simulink model "TestCinematiqueNew"  (Simulink 6.5)
settings: Solver=ode45  StartTime=0.0  StopTime=10.0  RelTol=1e-3
undefined symbols (not defined in the file): EngineSpeedTest, EngineSpeedTimeTest, x
settings Model: Creator=a030141  LastModifiedBy=Zeus
settings DataIOCC: SignalLoggingName=sigsOut
settings DebuggingCC: SolverPrmCheckMsg=none  MultiTaskDSMMsg=warning  MultiTaskCondExecSysMsg=none  StrictBusMsg=None
settings HardwareCC: TargetUnknown=on
settings RTWCC: IncludeERTFirstTime=on

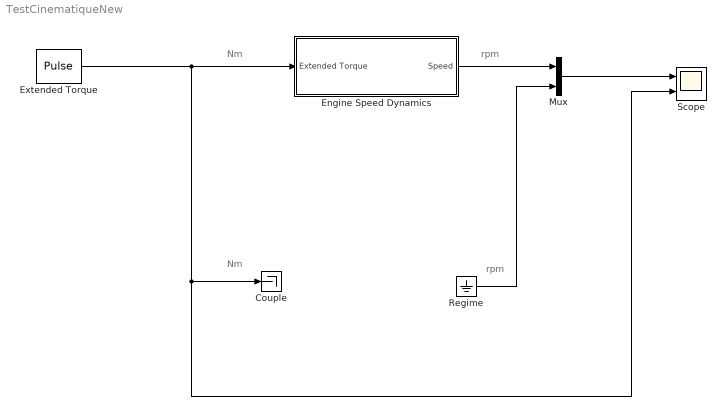
== system TestCinematiqueNew ==
  note: rpm
  note: rpm
  note: Nm
  note: Nm
  Couple : Terminator
  Engine Speed Dynamics : Subsystem
  Extended Torque : DiscretePulseGenerator  PulseType=Time based  PulseWidth=50
  Mux : Mux  Inputs=2
  Regime : Ground
  Scope : Scope  NumInputPorts=2
      settings: YMin=-5~-5  YMax=5~5
  wires:
  Extended Torque/1 -> Engine Speed Dynamics/1(Extended Torque), Scope/2, Couple/1
  Engine Speed Dynamics/1(Speed) -> Mux/1
  Mux/1 -> Scope/1
  Regime/1 -> Mux/2

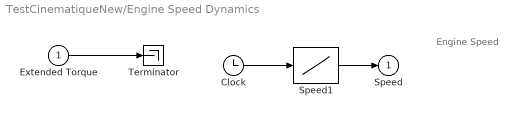
== system TestCinematiqueNew/Engine Speed Dynamics ==
  note: Engine Speed
  Extended Torque : Inport
  Clock : Clock
      settings: Decimation=10
  Speed1 : Lookup  InputValues=EngineSpeedTimeTest  OutputValues=EngineSpeedTest  LookUpMeth=Interpolation-Extrapolation  OutDataType=sfix(16)  OutScaling=2^0  SaturateOnIntegerOverflow=on  SampleTime=-1  LUTDesignTableMode=Redesign Table  LUTDesignDataSource=Block Dialog  LUTDesignFunctionName=sqrt(x)  LUTDesignUseExistingBP=on  LUTDesignRelError=0.01  LUTDesignAbsError=1e-6  RndMeth=Floor
      settings: LockScale=off
  Terminator : Terminator
  Speed : Outport
  wires:
  Speed1/1 -> Speed/1
  Clock/1 -> Speed1/1
  Extended Torque/1 -> Terminator/1
